simulink model "tracking"  (R2022a)
settings: Solver=VariableStepAuto  StartTime=0.0  StopTime=Traj.duration  FixedStep=0.0001  RelTol=1e-3  AbsTol=1e-3  EnableMultiTasking=on
InitFcn:
  | run('parameters.m')
  | run('initBusObjects.m')
  | run('loadTrajectory.m')
settings Model: Creator=chrismailer  LastModifiedBy=Chris
settings SolverCC: AutoScaleAbsTol=off  NumberNewtonIterations=3  ZeroCrossAlgorithm=Adaptive  AlgebraicLoopSolver=TrustRegion  AutoInsertRateTranBlk=on
settings DataIOCC: LimitDataPoints=on  MaxDataPoints=10000
settings OptimizationCC: LifeSpan=inf
settings DebuggingCC: UnconnectedInputMsg=warning  UnconnectedOutputMsg=warning  UnconnectedLineMsg=warning  AllowSymbolicDim=off  SFUnexpectedBacktrackingDiag=warning  SFNoUnconditionalDefaultTransitionDiag=warning  SFExecutionAtInitializationDiag=none  SFMachineParentedDataDiag=warning  ArithmeticOperatorsInVariantConditions=warning
settings SFSimCC: SimUseLocalCustomCode=off  CustomCodeUndefinedFunction=UseInterfaceOnly
settings RTWCC: RTWUseLocalCustomCode=off  DLArmComputeVersion=19.05
settings CodeAppCC: StateflowObjectComments=on
settings GRTTargetCC: TargetLangStandard=C89/C90 (ANSI)
settings ConfigComp: CovMetricSettings=dw  CovSaveCumulativeToWorkspaceVar=on  CovSaveSingleToWorkspaceVar=on  CovExternalEMLEnable=off  CovSFcnEnable=off
settings SimscapeCC: SimscapeLogType=all  SimscapeLogSimulationStatistics=on  SimscapeLogDataHistory=10000
settings ExplorerConfigSet: InternalSimMechanicsExplorerSettings="<ExplorerConfiguration><canonicalview>default</canonicalview><AnimationSetting><BasePlaybackSpeed>1.0</BasePlaybackSpeed><PlaybackSpeedFactor>1.0</PlaybackSpeedFactor></AnimationSetting><TilePanel><TileInfo><Tiles Columns=\"1\" Count=\"1\" Rows=\"1\"><Column Weight=\"1\"/><Row Weight=\"1\"/><Tile Height=\"1\" Width=\"1\" X=\"0\" Y=\"0\"/></Tiles></TileInfo><SceneInfo><SceneViewer><BGColor><R>1</R><G>1</G><B>1</B></BGColor><Camera><DoPerspective>off</DoPerspective><Position><X>-0.0041343314439558727</X><Y>-1.11921434473283221</Y><Z>0.175628602427760266</Z></Position><Center><X>-0.0041343314439558727</X><Y>-4.83918898563917566e-08</Y><Z>0.175628602427760266</Z></Center><Up><X>0</X><Y>-0</Y><Z>1</Z></Up><ViewLimDist>1</ViewLimDist><YLim>0.270059474200909144</YLim><XLim>0.399043103670000066</XLim></Camera></SceneViewer></SceneInfo></TilePanel><MechEditorPanel><Cameras/><GfxPanelCameraMap/><VideoCreator><PlaybackSpeedRatio>1.0</PlaybackSpeedRatio><FrameRate>30</FrameRate><VideoFormat>MPEG-4</VideoFormat><FrameSize>[1920 1080]</FrameSize></VideoCreator></MechEditorPanel></ExplorerConfiguration>"

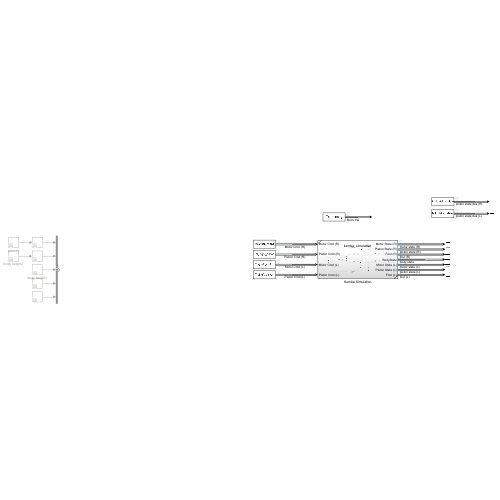
[thumbnail: Simulink's stored preview of the top-level diagram]
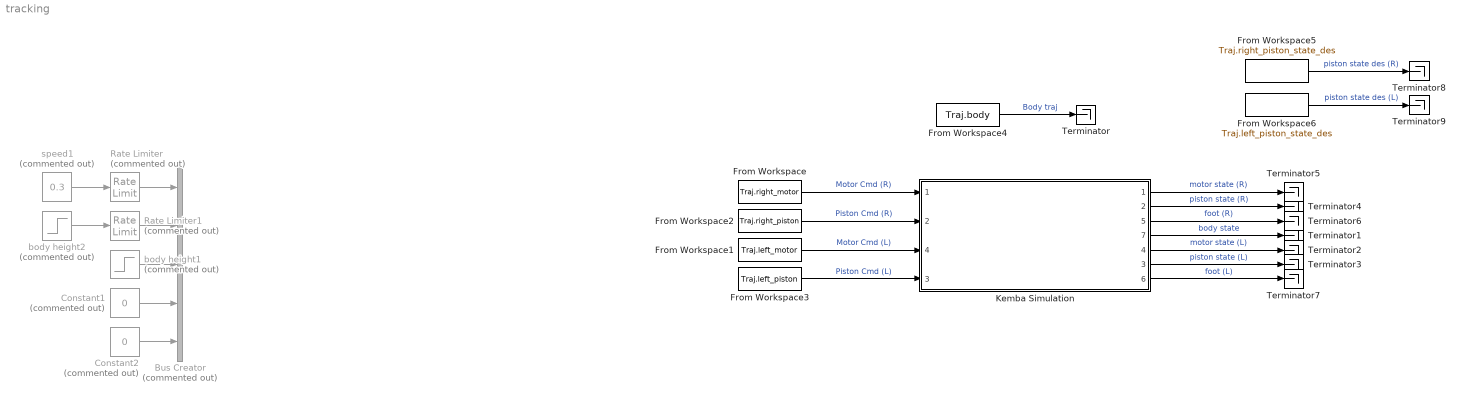
== system tracking ==
  Bus Creator : BusCreator  Commented=on  Inputs=5  OutDataTypeStr=Bus: Command
      settings: InheritFromInputs=off
  Constant1 : Constant  Commented=on  Value=0
  Constant2 : Constant  Commented=on  Value=0
  From Workspace : FromWorkspace  VariableName=Traj.right_motor  OutDataTypeStr=Bus: MotorCmd  SampleTime=0.001  Interpolate=off  OutputAfterFinalValue=Holding final value
  From Workspace1 : FromWorkspace  VariableName=Traj.left_motor  OutDataTypeStr=Bus: MotorCmd  SampleTime=0.001  Interpolate=off  OutputAfterFinalValue=Holding final value
  From Workspace2 : FromWorkspace  VariableName=Traj.right_piston  OutDataTypeStr=Bus: PistonCmd  SampleTime=0.001  Interpolate=off  OutputAfterFinalValue=Setting to zero
  From Workspace3 : FromWorkspace  VariableName=Traj.left_piston  OutDataTypeStr=Bus: PistonCmd  SampleTime=0.001  Interpolate=off  OutputAfterFinalValue=Setting to zero
  From Workspace4 : FromWorkspace  VariableName=Traj.body  OutDataTypeStr=Bus: BodyState  SampleTime=0.001  Interpolate=off  OutputAfterFinalValue=Holding final value
  From Workspace5 : FromWorkspace  VariableName=Traj.right_piston_state_des  OutDataTypeStr=Bus: PistonState  SampleTime=0.001  Interpolate=off  OutputAfterFinalValue=Holding final value
  From Workspace6 : FromWorkspace  VariableName=Traj.left_piston_state_des  OutDataTypeStr=Bus: PistonState  SampleTime=0.001  Interpolate=off  OutputAfterFinalValue=Holding final value
  Kemba Simulation : Subsystem  ReferencedSubsystem=kemba_simulation
      settings: PortSchema="{\"entries\":[{\"content\":{\"sides\":[{\"content\":{\"connectorIds\":[\"In1\",\"In2\",\"In4\",\"In3\"]},\"type\":\"ConnectorPlacement.EquallySpacedRectSide\",\"uuid\":\"35a785e7-99ad-4766-87e3-a239e5d8a8f8\"},{\"content\":{\"connectorIds\":[\"Out1\",\"Out2\",\"Out5\",\"Out7\",\"Out4\",\"Out3\",\"Out6\"],\"side\":\"RIGHT\"},\"type\":\"ConnectorPlacement.EquallySpacedRectSide\",\"uuid\":\"8c5f00f3-e1d5-4c02-a562-5da7bf8e4c30\"},{\"content\":{\"connectorIds\":[],\"side\":\"TOP\"},\"type\":\"ConnectorPlacement.EquallySpacedRectSide\",\"uuid\":\"cf7efd56-02a7-4dc2-b997-d6a0137d575f\"}]},\"type\":\"ConnectorPlacement.EquallySpacedConnector\",\"uuid\":\"7dd37b2d-e40a-4db8-86aa-8036efc7fb4f\"}],\"packageUris\":[\"http://schema.mathworks.com/mf0/Connector/R2020b\"],\"version\":\"1.0\"}"
  Rate Limiter : RateLimiter  Commented=on  RisingSlewLimit=0.05  FallingSlewLimit=-0.05  SampleTimeMode=inherited
  Rate Limiter1 : RateLimiter  Commented=on  RisingSlewLimit=0.2  FallingSlewLimit=-0.2  SampleTimeMode=inherited
  Terminator{,1..9} (10 alike) : Terminator
  body height1 : Step  Commented=on  Time=2  SampleTime=0
  body height2 : Step  Commented=on  Time=3  After=2  SampleTime=0
  speed1 : Constant  Commented=on  Value=0.3
  wires:
  Kemba Simulation/7 -> Terminator1/1  "body state"
  speed1/1 -> Rate Limiter/1
  Kemba Simulation/2 -> Terminator4/1  "piston state (R)"
  Kemba Simulation/1 -> Terminator5/1  "motor state (R)"
  Kemba Simulation/3 -> Terminator3/1  "piston state (L)"
  Kemba Simulation/4 -> Terminator2/1  "motor state (L)"
  body height1/1 -> Bus Creator/3
  From Workspace/1 -> Kemba Simulation/1  "Motor Cmd (R)"
  From Workspace2/1 -> Kemba Simulation/2  "Piston Cmd (R)"
  Kemba Simulation/5 -> Terminator6/1  "foot (R)"
  Kemba Simulation/6 -> Terminator7/1  "foot (L)"
  Rate Limiter/1 -> Bus Creator/1
  Constant2/1 -> Bus Creator/5
  Constant1/1 -> Bus Creator/4
  body height2/1 -> Rate Limiter1/1
  Rate Limiter1/1 -> Bus Creator/2
  From Workspace1/1 -> Kemba Simulation/4  "Motor Cmd (L)"
  From Workspace3/1 -> Kemba Simulation/3  "Piston Cmd (L)"
  From Workspace4/1 -> Terminator/1  "Body traj"
  From Workspace5/1 -> Terminator8/1  "piston state des (R)"
  From Workspace6/1 -> Terminator9/1  "piston state des (L)"
